simulink model "Dynamic_Leg_Model_2"  (R2018b)
settings: Solver=ode45  StartTime=0.0  StopTime=100.0  MaxStep=0.1  RelTol=1e-3
libraries: simulink x2
settings Model: Creator=jabyrns2  LastModifiedBy=jabyrns2
settings DebuggingCC: UnderSpecifiedDimensionMsg=warning

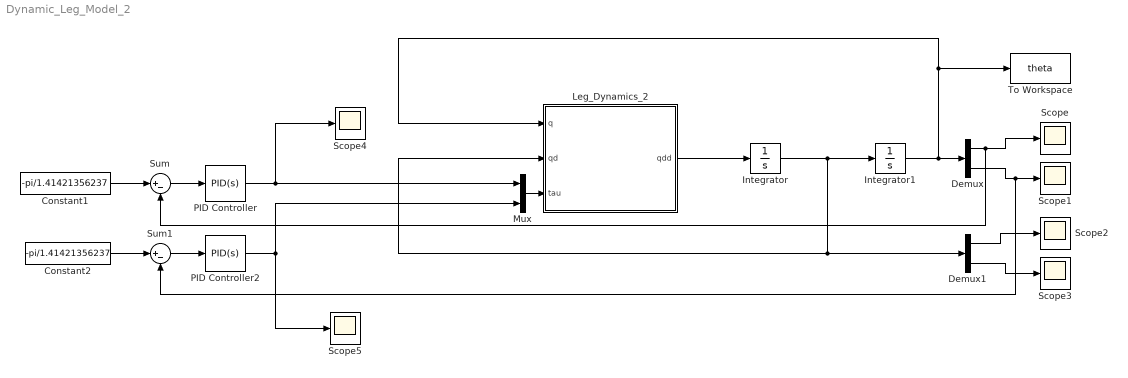
== system Dynamic_Leg_Model_2 ==
  Constant1 : Constant  Value=-pi/1.41421356237
  Constant2 : Constant  Value=-pi/1.41421356237
  Demux : Demux  Outputs=2
  Demux1 : Demux  Outputs=2
  Integrator : Integrator  InitialCondition=[0;0]
  Integrator1 : Integrator  InitialCondition=[-pi/1.41421356237;-pi/1.41421356237]
  Leg_Dynamics_2 : MATLAB Function  TreatAsAtomicUnit=on
  Mux : Mux  Inputs=2
  PID Controller : simulink/Continuous/PID Controller  Controller=PID  Form=Parallel  TimeDomain=Continuous-time  SampleTime=-1  IntegratorMethod=Forward Euler  FilterMethod=Forward Euler  ControllerParametersSource=internal  P=1.5  I=0.005  D=0.05  UseFilter=on  N=100  TunerSelectOption=Transfer Function Based (PID Tuner App)  InitialConditionSource=internal  InitialConditionForIntegrator=0  InitialConditionForFilter=0  DifferentiatorICPrevScaledInput=0  ExternalReset=none  TrackingMode=off  Kt=1  LimitOutput=off  UpperSaturationLimit=inf  LowerSaturationLimit=-inf  LinearizeAsGain=on  AntiWindupMode=none  Kb=1  POutMin=[]  POutMax=[]  IOutMin=[]  IOutMax=[]  DOutMin=[]  DOutMax=[]  NOutMin=[]  NOutMax=[]  SumOutMin=[]  SumOutMax=[]  SaturationOutMin=[]  SaturationOutMax=[]  PParamMin=[]  PParamMax=[]  IParamMin=[]  IParamMax=[]  DParamMin=[]  DParamMax=[]  NParamMin=[]  NParamMax=[]  KbParamMin=[]  KbParamMax=[]  KtParamMin=[]  KtParamMax=[]  KbOutMin=[]  KbOutMax=[]  KtOutMin=[]  KtOutMax=[]  IntegratorOutMin=[]  IntegratorOutMax=[]  FilterOutMin=[]  FilterOutMax=[]  SumI1OutMin=[]  SumI1OutMax=[]  SumI2OutMin=[]  SumI2OutMax=[]  SumI3OutMin=[]  SumI3OutMax=[]  SumI4OutMin=[]  SumI4OutMax=[]  SumDOutMin=[]  SumDOutMax=[]  DifferentiatorOutMin=[]  DifferentiatorOutMax=[]  FilterDiffOutCoefMin=[]  FilterDiffOutCoefMax=[]  ReciprocalOutMin=[]  ReciprocalOutMax=[]  SumDenOutMin=[]  SumDenOutMax=[]  SumNumOutMin=[]  SumNumOutMax=[]  DivideOutMin=[]  DivideOutMax=[]  IntegratorContinuousStateAttributes=''  IntegratorStateMustResolveToSignalObject=off  IntegratorRTWStateStorageClass=Auto  FilterContinuousStateAttributes=''  FilterStateMustResolveToSignalObject=off  FilterRTWStateStorageClass=Auto  ParallelPVariant=InternalParameters  IdealPVariant=Disabled  IVariant=InternalParameters  DVariant=InternalParameters  IntegratorVariant=Continuous  SatVariant=Disabled  AWVariant=Passthrough  PCopyVariant=Disabled  TRVariant=Disabled  FdbkBlocksVariant=Forward  IdealPFdbkVariant=Disabled  SatFdbkVariant=Disabled  DerivativeFilterVariant=ContFilter  NVariant=InternalParameters  NCopyVariant=Disabled  FilterICVariant=InternalICsFilter  IntegratorICVariant=InternalICs  ExternalResetVariant=Disabled  TRSumVariant=Passthrough  SumFdbkVariant=Disabled  SumVariant=Sum_PID
  PID Controller2 : simulink/Continuous/PID Controller  Controller=PID  Form=Parallel  TimeDomain=Continuous-time  SampleTime=-1  IntegratorMethod=Forward Euler  FilterMethod=Forward Euler  ControllerParametersSource=internal  P=1.5  I=0.005  D=0.05  UseFilter=on  N=100  TunerSelectOption=Transfer Function Based (PID Tuner App)  InitialConditionSource=internal  InitialConditionForIntegrator=0  InitialConditionForFilter=0  DifferentiatorICPrevScaledInput=0  ExternalReset=none  TrackingMode=off  Kt=1  LimitOutput=off  UpperSaturationLimit=inf  LowerSaturationLimit=-inf  LinearizeAsGain=on  AntiWindupMode=none  Kb=1  POutMin=[]  POutMax=[]  IOutMin=[]  IOutMax=[]  DOutMin=[]  DOutMax=[]  NOutMin=[]  NOutMax=[]  SumOutMin=[]  SumOutMax=[]  SaturationOutMin=[]  SaturationOutMax=[]  PParamMin=[]  PParamMax=[]  IParamMin=[]  IParamMax=[]  DParamMin=[]  DParamMax=[]  NParamMin=[]  NParamMax=[]  KbParamMin=[]  KbParamMax=[]  KtParamMin=[]  KtParamMax=[]  KbOutMin=[]  KbOutMax=[]  KtOutMin=[]  KtOutMax=[]  IntegratorOutMin=[]  IntegratorOutMax=[]  FilterOutMin=[]  FilterOutMax=[]  SumI1OutMin=[]  SumI1OutMax=[]  SumI2OutMin=[]  SumI2OutMax=[]  SumI3OutMin=[]  SumI3OutMax=[]  SumI4OutMin=[]  SumI4OutMax=[]  SumDOutMin=[]  SumDOutMax=[]  DifferentiatorOutMin=[]  DifferentiatorOutMax=[]  FilterDiffOutCoefMin=[]  FilterDiffOutCoefMax=[]  ReciprocalOutMin=[]  ReciprocalOutMax=[]  SumDenOutMin=[]  SumDenOutMax=[]  SumNumOutMin=[]  SumNumOutMax=[]  DivideOutMin=[]  DivideOutMax=[]  IntegratorContinuousStateAttributes=''  IntegratorStateMustResolveToSignalObject=off  IntegratorRTWStateStorageClass=Auto  FilterContinuousStateAttributes=''  FilterStateMustResolveToSignalObject=off  FilterRTWStateStorageClass=Auto  ParallelPVariant=InternalParameters  IdealPVariant=Disabled  IVariant=InternalParameters  DVariant=InternalParameters  IntegratorVariant=Continuous  SatVariant=Disabled  AWVariant=Passthrough  PCopyVariant=Disabled  TRVariant=Disabled  FdbkBlocksVariant=Forward  IdealPFdbkVariant=Disabled  SatFdbkVariant=Disabled  DerivativeFilterVariant=ContFilter  NVariant=InternalParameters  NCopyVariant=Disabled  FilterICVariant=InternalICsFilter  IntegratorICVariant=InternalICs  ExternalResetVariant=Disabled  TRSumVariant=Passthrough  SumFdbkVariant=Disabled  SumVariant=Sum_PID
  Scope{,1..5} (6 alike) : Scope
  Sum : Sum  Inputs=|+-
  Sum1 : Sum  Inputs=|+-
  To Workspace : ToWorkspace  VariableName=theta  SampleTime=-1
  wires:
  Integrator/1 -> Demux1/1, Leg_Dynamics_2/2(qd), Integrator1/1
  Integrator1/1 -> To Workspace/1, Leg_Dynamics_2/1(q), Demux/1
  Demux/1 -> Scope/1, Sum/2
  Demux/2 -> Scope1/1, Sum1/2
  Demux1/1 -> Scope2/1
  Demux1/2 -> Scope3/1
  Mux/1 -> Leg_Dynamics_2/3(tau)
  PID Controller/1 -> Mux/1, Scope4/1
  PID Controller2/1 -> Scope5/1, Mux/2
  Leg_Dynamics_2/1(qdd) -> Integrator/1
  Constant1/1 -> Sum/1
  Sum/1 -> PID Controller/1
  Constant2/1 -> Sum1/1
  Sum1/1 -> PID Controller2/1

== matlab function Dynamic_Leg_Model_2/Leg_Dynamics_2 ==
  data: q input; qdd output; qd input; tau input
function qdd = Leg_Dynamics_2(q, qd, tau)
    t1 = q(1);
    t2 = q(2);
    t1d = qd(1);
    t2d = qd(2);
    tau1 = tau(1);
    tau2 = tau(2);

    l1 = 0.215; % 215mm
    l2 = 0.215; % 215mm
    lc1 = 0.1; % 100mm ---CHANGE
    lc2 = 0.215; % 215mm  ---CHANGE
    m1 = 0.132; % 950 grams ---CHANGE
    m2 = 0.941; % 100 grams ---CHANGE
    i1 = 0.01;
    i2 = 0.5;

    p1 = m1*lc1 + m2*lc1*lc1 + i1;
    p2 = m2*lc2*lc2 + i2;
    p3 = m2*l1*lc2;
    p4 = m1*lc1*m2*l1;
    p5 = m2*lc2;

    D = [p1 + p2 + 2*p3*cos(t2) , p2 + p3*cos(t2); p2 + p3*cos(t2) , p2];

    C = [-p3*sin(t2)*t2d , -p3*sin(t2)*t2d - p3*sin(t2)*t1d; p3*sin(t2)*t1d , 0];

    G = [-p4*(-9.81)*cos(t1) - p5*(-9.81)*cos(t1 + t2) ; -p5*(-9.81)*cos(t1 + t2)];
    
    qdd = inv(D)*[tau1;tau2]-inv(D)*C*qd - inv(D)*G;
end
